simulink model "PIDController_theta4"  (R2022a)
settings: Solver=ode5  StartTime=0.0  StopTime=0.0019831  FixedStep=4.9578e-05  RelTol=1e-3
settings Model: Creator=Admin  LastModifiedBy=mquyet
settings SolverCC: AlgebraicLoopSolver=TrustRegion
settings DataIOCC: ReturnWorkspaceOutputs=off
settings DebuggingCC: UnconnectedInputMsg=warning  UnconnectedOutputMsg=warning  UnconnectedLineMsg=warning  SFMachineParentedDataDiag=warning  ArithmeticOperatorsInVariantConditions=warning
settings SFSimCC: SimUseLocalCustomCode=off  CustomCodeUndefinedFunction=UseInterfaceOnly
settings RTWCC: RTWUseLocalCustomCode=off
settings CodeAppCC: StateflowObjectComments=on

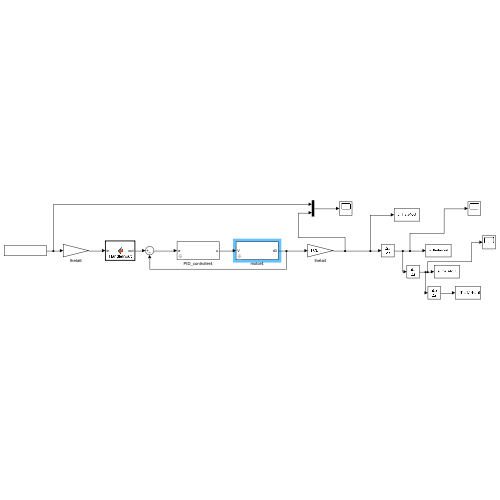
[thumbnail: Simulink's stored preview of the top-level diagram]
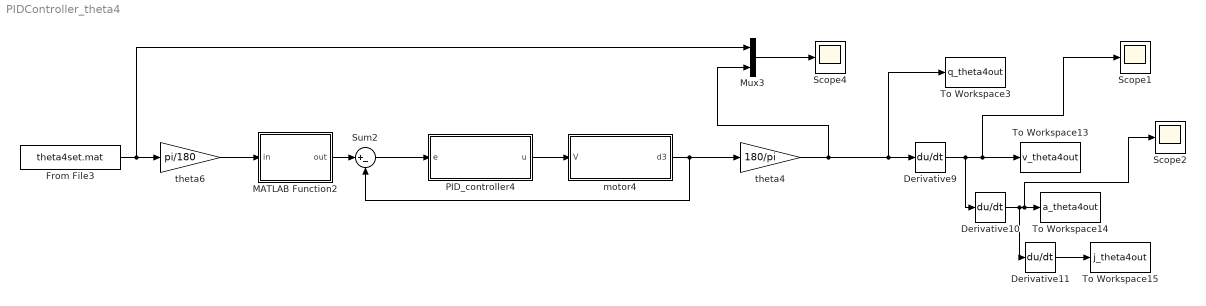
== system PIDController_theta4 ==
  Derivative10 : Derivative
  Derivative11 : Derivative
  Derivative9 : Derivative
  From File3 : FromFile  FileName=theta4set.mat
  MATLAB Function2 : MATLAB Function  TreatAsAtomicUnit=on
  Mux3 : Mux  Inputs=2
  PID_controller4 : Subsystem  mask{Kp=10000, Ki=0, Kd=100}
  Scope1 : Scope
  Scope2 : Scope
  Scope4 : Scope
  Sum2 : Sum  Inputs=|+-
  To Workspace13 : ToWorkspace  VariableName=v_theta4out  SampleTime=-1
  To Workspace14 : ToWorkspace  VariableName=a_theta4out  SampleTime=-1
  To Workspace15 : ToWorkspace  VariableName=j_theta4out  SampleTime=-1
  To Workspace3 : ToWorkspace  VariableName=q_theta4out  SampleTime=-1
  motor4 : Subsystem  mask{Ki=0.1, Kb=0.1, L=0.5, R=2, Jeff=0.02, Beff=0.2, N=100}
  theta4 : Gain  Gain=180/pi
  theta6 : Gain  Gain=pi/180
  wires:
  From File3/1 -> Mux3/1, theta6/1
  MATLAB Function2/1(out) -> Sum2/1
  theta4/1 -> Mux3/2, Derivative9/1, To Workspace3/1
  Derivative9/1 -> Derivative10/1, Scope1/1, To Workspace13/1
  Derivative10/1 -> Derivative11/1, Scope2/1, To Workspace14/1
  Derivative11/1 -> To Workspace15/1
  theta6/1 -> MATLAB Function2/1(in)
  Mux3/1 -> Scope4/1
  motor4/1(d3) -> theta4/1, Sum2/2
  PID_controller4/1(u) -> motor4/1(V)
  Sum2/1 -> PID_controller4/1(e)

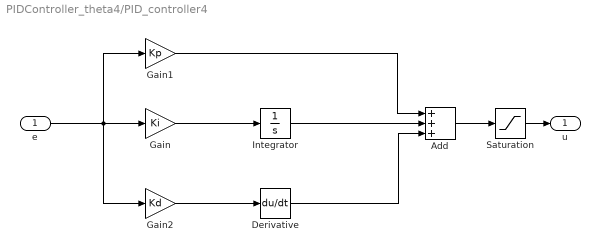
== system PIDController_theta4/PID_controller4 ==
  e : Inport
  Add : Sum  Inputs=+++
  Derivative : Derivative
  Gain : Gain  Gain=Ki
  Gain1 : Gain  Gain=Kp
  Gain2 : Gain  Gain=Kd
  Integrator : Integrator
  Saturation : Saturate  UpperLimit=300  LowerLimit=-300
  u : Outport  VectorParamsAs1DForOutWhenUnconnected=off
  wires:
  e/1 -> Gain2/1, Gain1/1, Gain/1
  Gain/1 -> Integrator/1
  Gain2/1 -> Derivative/1
  Gain1/1 -> Add/1
  Integrator/1 -> Add/2
  Derivative/1 -> Add/3
  Add/1 -> Saturation/1
  Saturation/1 -> u/1

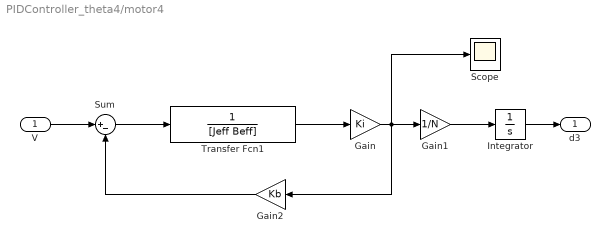
== system PIDController_theta4/motor4 ==
  V : Inport
  Gain : Gain  Gain=Ki
  Gain1 : Gain  Gain=1/N
  Gain2 : Gain  Gain=Kb
  Integrator : Integrator  InitialCondition=40.6737
  Scope : Scope
  Sum : Sum  Inputs=|+-
  Transfer Fcn1 : TransferFcn  Denominator=[Jeff Beff]
  d3 : Outport  VectorParamsAs1DForOutWhenUnconnected=off
  wires:
  Transfer Fcn1/1 -> Gain/1
  Gain1/1 -> Integrator/1
  Integrator/1 -> d3/1
  Gain2/1 -> Sum/2
  V/1 -> Sum/1
  Sum/1 -> Transfer Fcn1/1
  Gain/1 -> Gain1/1, Gain2/1, Scope/1

== matlab function PIDController_theta4/MATLAB Function2 ==
  settings: updateMethod=DISCRETE
  data: in input; out output
function out = HandleInput(in)

out = in;
persistent pre
if isempty(pre)
    pre = 0;
end

while (out - pre > 1.5*pi)
    out = out - 2*pi;
end

while (out - pre < -1.5*pi)
    out = out + 2*pi;
end
